simulink model "lab7step"  (R2015b)
settings: Solver=ode4  StartTime=0.0  StopTime=4  FixedStep=0.002  RelTol=1e-3
values from neighbouring files (symbols this model uses):
  alpha = 1/K(1)    [lab05.m]
  K1 = (r-1)*wn^3/(2*z*a)    [lab06.m]
  Kd = (((2*z*wn)-tau +(((r-1)*wn)/(2*z)))/a)    [lab06.m]
  Kg = KgHigh    (= 70)    [lab05.m]
  Kp = (r/a)*wn^2    [lab06.m]
  tau = K(2)*alpha    [lab05.m]
undefined symbols (not defined in the file or in its folder): HIL, qc_get_step_size
libraries: quarc_library x4
settings Model: SimulationMode=external  ExtModeTrigDuration=10000  Creator=husseinz  LastModifiedBy=dilsizk
settings SolverCC: PositivePriorityOrder=on
settings RTWCC: SystemTargetFile=quarc_win64.tlc  TemplateMakefile=quarc_default_tmf  Description=QUARC Win64 Target
settings STFCustomTargetCC: TargetPreCompLibLocation=C:\ProgramData\QUARC\lib\2015b\win64\release  GeneratePreprocessorConditionals=Use local settings  CPPClassGenCompliant=off
settings GRTTargetCC: TargetPreCompLibLocation=C:\ProgramData\QUARC\lib\2015b\win64\release  ParMdlRefBuildCompliant=off  CompOptLevelCompliant=off  CombineOutputUpdateFcns=off  MatFileLogging=off  CPPClassGenCompliant=off  GRTInterface=on  UseToolchainInfoCompliant=off  ExtMode=on  ExtModeMexFile=quarc_comm

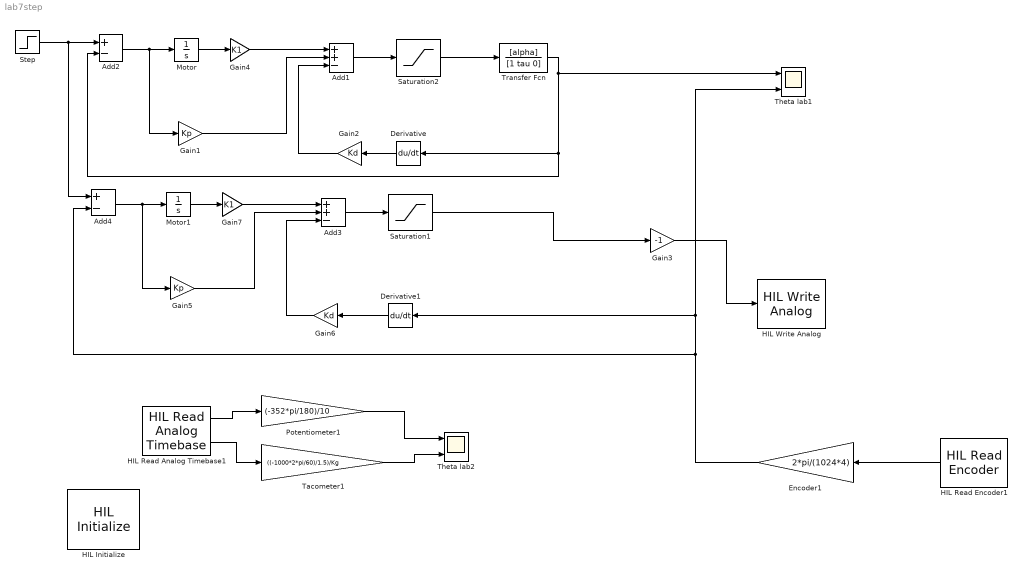
== system lab7step ==
  Add1 : Sum  Inputs=++-
  Add2 : Sum  Inputs=+-
  Add3 : Sum  Inputs=++-
  Add4 : Sum  Inputs=+-
  Derivative : Derivative
  Derivative1 : Derivative
  Encoder1 : Gain  Gain=2*pi/(1024*4)
  Gain1 : Gain  Gain=Kp
  Gain2 : Gain  Gain=Kd
  Gain3 : Gain  Gain=-1
  Gain4 : Gain  Gain=K1
  Gain5 : Gain  Gain=Kp
  Gain6 : Gain  Gain=Kd
  Gain7 : Gain  Gain=K1
  HIL Initialize : quarc_library/Data Acquisition/Generic/Configuration/HIL Initialize  Priority=-99  object_name=HIL-2  board_type=q8_usb  board_number=0  board_options=update_rate=normal;decimation=1  exclusive=off  active=off  hardware_clocks=[0:2]  clock_modes=[]  initial_clock_frequencies=[]  set_clock_params_at_start=off  set_clock_params_at_switch_in=off  set_clock_frequencies_at_start=off  set_clock_frequencies_at_switch_in=off  analog_input_channels=[0:7]  analog_input_maximums=10  analog_input_minimums=-10  set_analog_input_params_at_start=on  set_analog_input_params_at_switch_in=off  analog_output_channels=[0:7]  analog_output_maximums=10  analog_output_minimums=-10  initial_analog_outputs=[0]  final_analog_outputs=[0]  watchdog_analog_outputs=0  set_analog_output_params_at_start=on  set_analog_output_params_at_switch_in=off  set_analog_outputs_at_start=on  set_analog_outputs_at_switch_in=off  set_analog_outputs_at_terminate=on  set_analog_outputs_at_switch_out=off  set_analog_outputs_on_watchdog=off  digital_input_channels=[]  digital_output_channels=[]  digital_output_configuration=[]  initial_digital_outputs=[1]  final_digital_outputs=[1]  watchdog_digital_outputs=[1]  set_digital_output_params_at_start=off  set_digital_output_params_at_switch_in=off  set_digital_outputs_at_start=on  set_digital_outputs_at_switch_in=off  set_digital_outputs_at_terminate=on  set_digital_outputs_at_switch_out=off  set_digital_outputs_on_watchdog=off  encoder_channels=[0:7]  quadrature=[4]  encoder_filter_frequency=[]  initial_encoder_counts=[0]  set_encoder_params_at_start=on  set_encoder_params_at_switch_in=off  set_encoder_counts_at_start=on  set_encoder_counts_at_switch_in=off  pwm_channels=[0:7]  pwm_modes=0  pwm_frequency=99.532799999999995e6/4095  pwm_configuration=[0]  pwm_alignment=[0]  pwm_polarity=[1]  pwm_leading_deadband=[0]  pwm_trailing_deadband=[0]  initial_pwm_outputs=[0]  final_pwm_outputs=[0]  watchdog_pwm_outputs=[0]  set_pwm_params_at_start=on  set_pwm_params_at_switch_in=off  set_pwm_outputs_at_start=on  set_pwm_outputs_at_switch_in=off  set_pwm_outputs_at_terminate=on  set_pwm_outputs_at_switch_out=off  set_pwm_outputs_on_watchdog=off  other_output_channels=[]  initial_other_outputs=[]  final_other_outputs=[]  watchdog_other_outputs=[]  set_other_outputs_at_start=off  set_other_outputs_at_switch_in=off  set_other_outputs_at_terminate=off  set_other_outputs_at_switch_out=off  set_other_outputs_on_watchdog=off
  HIL Read Analog Timebase1 : quarc_library/Data Acquisition/Generic/Timebases/HIL Read Analog Timebase  object_name=HIL-2  clock=0  channels=[0:1]  samples_in_buffer=max(ceil(1/qc_get_step_size), 1)  active=on  vector_output=off
      settings: AttributesFormatString=(%<object_name>)
  HIL Read Encoder1 : quarc_library/Data Acquisition/Generic/Immediate I//O/HIL Read Encoder  object_name=HIL-2  channels=[0]  sample_time=qc_get_step_size  active=on  vector_output=off  data_type_mode=Inherit via back propagation  data_type=double
  HIL Write Analog : quarc_library/Data Acquisition/Generic/Immediate I//O/HIL Write Analog  object_name=HIL-2  channels=0  sample_time=-1  active=off  vector_input=off
  Motor : Integrator
  Motor1 : Integrator
  Potentiometer1 : Gain  Gain=(-352*pi/180)/10
  Saturation1 : Saturate  UpperLimit=10  LowerLimit=-10
  Saturation2 : Saturate  UpperLimit=10  LowerLimit=-10
  Step : Step  After=pi/2  SampleTime=0
  Tacometer1 : Gain  Gain=((-1000*2*pi/60)/1.5)/Kg
  Theta lab1 : Scope  NumInputPorts=2
  Theta lab2 : Scope  NumInputPorts=2
  Transfer Fcn : TransferFcn  Numerator=[alpha]  Denominator=[1 tau 0]
  wires:
  Add2/1 -> Gain1/1, Motor/1
  Motor/1 -> Gain4/1
  Gain1/1 -> Add1/2
  Gain4/1 -> Add1/1
  Gain2/1 -> Add1/3
  Derivative/1 -> Gain2/1
  Transfer Fcn/1 -> Theta lab1/1, Add2/2, Derivative/1
  Saturation2/1 -> Transfer Fcn/1
  Add1/1 -> Saturation2/1
  Gain3/1 -> HIL Write Analog/1
  Add4/1 -> Gain5/1, Motor1/1
  Motor1/1 -> Gain7/1
  Gain5/1 -> Add3/2
  Gain7/1 -> Add3/1
  Gain6/1 -> Add3/3
  Add3/1 -> Saturation1/1
  Saturation1/1 -> Gain3/1
  HIL Read Analog Timebase1/2 -> Tacometer1/1
  HIL Read Analog Timebase1/1 -> Potentiometer1/1
  HIL Read Encoder1/1 -> Encoder1/1
  Encoder1/1 -> Theta lab1/2, Derivative1/1, Add4/2
  Step/1 -> Add4/1, Add2/1
  Derivative1/1 -> Gain6/1
  Potentiometer1/1 -> Theta lab2/1
  Tacometer1/1 -> Theta lab2/2
